simulink library "ChimeSystemLib"  (R2022b)
settings: Solver=VariableStepAuto  StartTime=0.0  StopTime=10.0  RelTol=1e-3
values from neighbouring files (symbols this model uses):
  include_eq_for_external_chime = 0    [chimes_init.m]
undefined symbols (not defined in the file or in its folder): chimeConfig, sys_defs
libraries: ChimeSystemLibBtc x1
settings Model: Creator=nikunj.tapodhan  LastModifiedBy=kl13806
settings SolverCC: AlgebraicLoopSolver=TrustRegion
settings DebuggingCC: UnconnectedInputMsg=warning  UnconnectedOutputMsg=warning  UnconnectedLineMsg=warning  SFMachineParentedDataDiag=warning  ArithmeticOperatorsInVariantConditions=warning
settings ModelReferenceCC: EnableRefExpFcnMdlSchedulingChecks=on
settings SFSimCC: CustomCodeUndefinedFunction=UseInterfaceOnly
settings RTWCC: DLArmComputeVersion=19.05

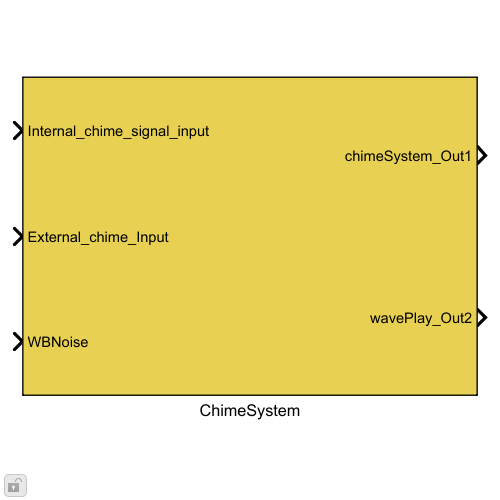
[thumbnail: Simulink's stored preview of the top-level diagram]
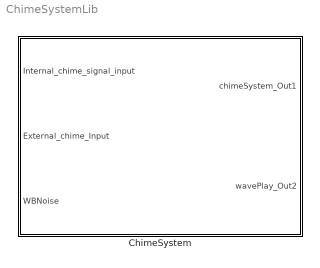
== system ChimeSystemLib ==
  ChimeSystem : Subsystem  mask{Fs_Hz=sys_defs.Fs_Hz, frameSize_samples=sys_defs.frameSize_samples, sineTableLength=sys_defs.sineTableLength, num_internal_chime=chimeConfig.scalarchime.num_internal_chime, num_external_chime=chimeConfig.ExternalChime.num_external_chime, num_click_clack=chimeConfig.scalarchime.num_click_clack, include_internal_chime_flag=chimeConfig.scalarchime.include_internal_chime_flag, include_external_chime_flag=chimeConfig.ExternalChime.include_external_chime_flag, nch=chimeConfig.scalarchime.nch, num_inp_chs=chimeConfig.scalarchime.num_inp_chs, NSTATES=chimeConfig.scalarchime.NSTATES, decrementVals=chimeConfig.scalarchime.decrementVals, count=chimeConfig.scalarchime.count, countDecrement=chimeConfig.scalarchime.countDecrement, state=chimeConfig.scalarchime.state, countState=chimeConfig.scalarchime.countState, nextState_expired=chimeConfig.scalarchime.nextState_expired, nextState_notExpired=chimeConfig.scalarchime.nextState_notExpired, outputState=chimeConfig.scalarchime.outputState, IDLE=chimeConfig.scalarchime.IDLE, RISE=chimeConfig.scalarchime.RISE, FALL=chimeConfig.scalarchime.FALL, CHECK_PULSE_COUNT=chimeConfig.scalarchime.CHECK_PULSE_COUNT, WAIT_FOR_PERIOD=chimeConfig.scalarchime.WAIT_FOR_PERIOD, CHECK_GROUP_COUNT=chimeConfig.scalarchime.CHECK_GROUP_COUNT, CHIMECONTROL_NSTATES=chimeConfig.scalarchime.CHIMECONTROL_NSTATES, volume=chimeConfig.scalarchime.volume, riseTime=chimeConfig.scalarchime.riseTime, onTime=chimeConfig.scalarchime.onTime, fallTime=chimeConfig.scalarchime.fallTime, offTime=chimeConfig.scalarchime.offTime, numPulses=chimeConfig.scalarchime.numPulses, period=chimeConfig.scalarchime.period, startOfFinalChime=chimeConfig.scalarchime.startOfFinalChime, endOfFinalChime=chimeConfig.scalarchime.endOfFinalChime, chimeEndNotification=chimeConfig.scalarchime.chimeEndNotification, newProfile=chimeConfig.scalarchime.newProfile, chimeRouting=chimeConfig.scalarchime.chimeRouting, num_chime_count=chimeConfig.scalarchime.num_chime_count, chime_group_count=chimeConfig.scalarchime.chime_group_count, spkrRouting=chimeConfig.scalarchime.spkrRouting, chimePlayPending=chimeConfig.scalarchime.chimePlayPending, remainingCount=chimeConfig.scalarchime.remainingCount, FW_AppendHostNotification=chimeConfig.scalarchime.FW_AppendHostNotification, chimeCancel=chimeConfig.scalarchime.chimeCancel, chimeType=chimeConfig.scalarchime.chimeType, nInternalBeepsGongs=sys_defs.nInternalBeepsGongs, chime_input_index=chimeConfig.scalarchime.chime_input_index, include_internal_click_clack=chimeConfig.scalarchime.include_internal_click_clack, thresholdNumPulse=chimeConfig.scalarchime.thresholdNumPulse, playControl=chimeConfig.wplay.playControl, include_eq_for_external_chime=include_eq_for_external_chime, OffsetIntChime=chimeConfig.scalarchime.OffsetIntChime, SelectNumIntChimes=chimeConfig.scalarchime.SelectNumIntChimes, immediately=chimeConfig.scalarchime.immediately, forever=chimeConfig.scalarchime.forever, playback_flag=chimeConfig.scalarchime.playback_flag, sysin_channel_count=chimeConfig.rgainz.sysin_channel_count, gain=chimeConfig.rgainz.gain, initial_linear_gain=chimeConfig.ExternalChime.TargetGainVal, nIn=chimeConfig.chimeRouter.In, output_index=chimeConfig.chimeRouter.output_indxs, len=chimeConfig.wplay.len, table=chimeConfig.wplay.table, tableIndex=chimeConfig.wplay.tableIndex, controlState=chimeConfig.wplay.controlState, minVol=chimeConfig.wplay.minVol, externalChimeCancel=chimeConfig.ExternalChime.externalChimeCancel}
      mask prompts: num_external_chime "NumberOfExternalChimeSignal"; sysin_channel_count "Number_of_rampers"; gain "Initial ramper gains"; initial_linear_gain "InitialRamperGainForExternalChime"; nIn "ChannelForChimeRouter"; output_index "ChannelIndexForChimeRouter"; len "WavePlay_len"; table "WavePlay_table"; tableIndex "WavePlay_tableIndex"; controlState "WavePlay_controlState"; minVol "WavePlay_minVol"
      mask init:
      | blkh = gcbh;
      | % Copy discrete mask parameters into a classdef object
      | InnerLinkConfig = ChimeSystemConfig;
      | InnerLinkConfig.FsHz = Fs_Hz;
      | InnerLinkConfig.FrameSizeSamples = frameSize_samples;
      | InnerLinkConfig.SineTableLength = sineTableLength;
      | InnerLinkConfig.NumInternalChime = num_internal_chime;
      | InnerLinkConfig.NumExternalChime = num_external_chime;
      | InnerLinkConfig.NumClickClack = num_click_clack;
      | InnerLinkConfig.IncludeInternalChimeFlag = include_internal_chime_flag;
      | %InnerLinkConfig.IncludeExternalChimeFlag = include_external_chime_flag;
      | InnerLinkConfig.Nch = nch;
      | InnerLinkConfig.NumInpChs = num_inp_chs;
      | InnerLinkConfig.NStates = NSTATES;
      | InnerLinkConfig.DecrementVals = decrementVals;
      | InnerLinkConfig.Count = count;
      | InnerLinkConfig.CountDecrement = countDecrement;
      | InnerLinkConfig.State = state;
      | InnerLinkConfig.CountState = countState;
      | InnerLinkConfig.NextStateExpired = nextState_expired;
      | InnerLinkConfig.NextStateNotExpired = nextState_notExpired;
      | InnerLinkConfig.OutputState = outputState;
      | InnerLinkConfig.Idle = IDLE;
      | InnerLinkConfig.Rise = RISE;
      | InnerLinkConfig.Fall = FALL;
      | InnerLinkConfig.CheckPulseCount = CHECK_PULSE_COUNT;
      | InnerLinkConfig.WaitForPeriod = WAIT_FOR_PERIOD;
      | InnerLinkConfig.CheckGroupCount = CHECK_GROUP_COUNT;
      | InnerLinkConfig.ChimecontrolNstates = CHIMECONTROL_NSTATES;
      | InnerLinkConfig.Volume = volume;
      | InnerLinkConfig.RiseTime = riseTime;
      | InnerLinkConfig.OnTime = onTime;
      | InnerLinkConfig.FallTime = fallTime;
      | InnerLinkConfig.OffTime = offTime;
      | InnerLinkConfig.NumPulses = numPulses;
      | InnerLinkConfig.Period = period;
      | InnerLinkConfig.StartOfFinalChime = startOfFinalChime;
      | InnerLinkConfig.EndOfFinalChime = endOfFinalChime;
      | InnerLinkConfig.ChimeEndNotification = chimeEndNotification;
      | InnerLinkConfig.NewProfile = newProfile;
      | InnerLinkConfig.ChimeRouting = chimeRouting;
      | InnerLinkConfig.NumChimeCount = num_chime_count;
      | InnerLinkConfig.ChimeGroupCount = chime_group_count;
      | InnerLinkConfig.SpkrRouting = spkrRouting;
      | InnerLinkConfig.ChimePlayPending = chimePlayPending;
      | InnerLinkConfig.RemainingCount = remainingCount;
      | InnerLinkConfig.FwAppendHostNotification = FW_AppendHostNotification;
      | InnerLinkConfig.ChimeCancel = chimeCancel;
      | InnerLinkConfig.ChimeType = chimeType;
      | InnerLinkConfig.NInternalBeepsGongs = nInternalBeepsGongs;
      | InnerLinkConfig.ChimeInputIndex = chime_input_index;
      | InnerLinkConfig.IncludeInternalClickClack = include_internal_click_clack;
      | InnerLinkConfig.ThresholdNumPulse = thresholdNumPulse;
      | InnerLinkConfig.PlayControl = playControl;
      | %InnerLinkConfig.IncludeEqForExternalChime = include_eq_for_external_chime;
      | InnerLinkConfig.OffsetIntChime = OffsetIntChime;
      | InnerLinkConfig.SelectNumIntChimes = SelectNumIntChimes;
      | InnerLinkConfig.Immediately = immediately;
      | InnerLinkConfig.Forever = forever;
      | InnerLinkConfig.PlaybackFlag = playback_flag;
      | InnerLinkConfig.SysinChannelCount = sysin_channel_count;
      | InnerLinkConfig.Gain = gain;
      | % InnerLinkConfig.InitialLinearGain = initial_linear_gain;
      | % InnerLinkConfig.NIn = nIn;
      | % InnerLinkConfig.OutputIndex = output_index;
      | InnerLinkConfig.Len = len;
      | % InnerLinkConfig.Table = table;
      | InnerLinkConfig.TableIndex = tableIndex;
      | % InnerLinkConfig.ControlState = controlState;
      | InnerLinkConfig.MinVol = minVol;
      | InnerLinkConfig.ExternalChimeCancel = externalChimeCancel;

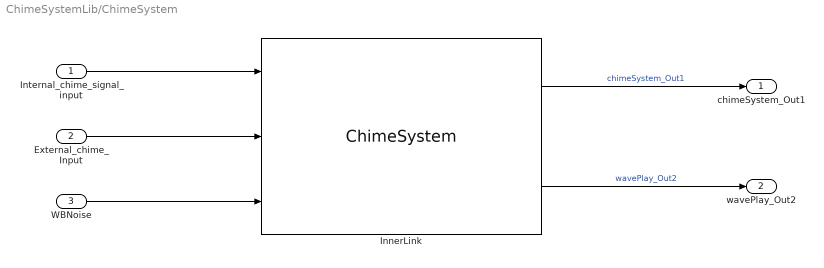
== system ChimeSystemLib/ChimeSystem ==
  Internal_chime_signal_input : Inport
  External_chime_Input : Inport  Port=2
  WBNoise : Inport  Port=3
  InnerLink : ChimeSystemLibBtc/ChimeSystem  Config=InnerLinkConfig
      settings: SourceProductName=Bose Blocklib
  chimeSystem_Out1 : Outport
  wavePlay_Out2 : Outport  Port=2
  wires:
  InnerLink/1 -> chimeSystem_Out1/1  "chimeSystem_Out1"
  InnerLink/2 -> wavePlay_Out2/1  "wavePlay_Out2"
  Internal_chime_signal_input/1 -> InnerLink/1
  External_chime_Input/1 -> InnerLink/2
  WBNoise/1 -> InnerLink/3
